simulink model "SUBS_PERFIL_OBSTACULOS"  (R2024b)
settings: Solver=VariableStepAuto  StartTime=0.0  StopTime=10.0  RelTol=1e-3
undefined symbols (not defined in the file): Wc
settings Model: Creator=juani  LastModifiedBy=juani

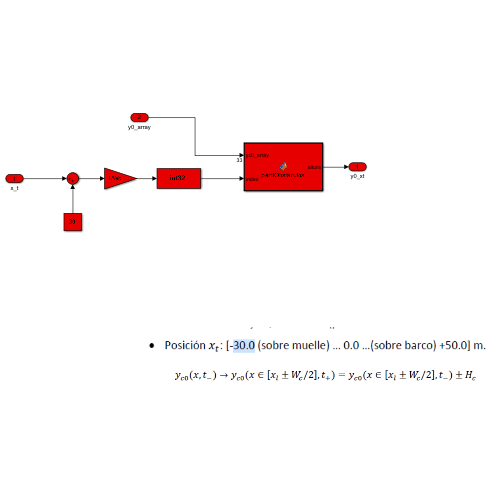
[thumbnail: Simulink's stored preview of the top-level diagram]
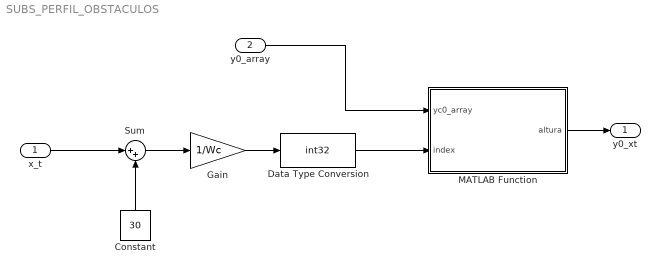
== system SUBS_PERFIL_OBSTACULOS ==
  x_t : Inport
  y0_array : Inport  Port=2
  Constant : Constant  Value=30
  Data Type Conversion : DataTypeConversion  OutDataTypeStr=int32  SaturateOnIntegerOverflow=off  RndMeth=Floor
  Gain : Gain  Gain=1/Wc
  MATLAB Function : MATLAB Function  TreatAsAtomicUnit=on
  Sum : Sum  Inputs=|++
  y0_xt : Outport
  wires:
  x_t/1 -> Sum/1
  Constant/1 -> Sum/2
  Sum/1 -> Gain/1
  y0_array/1 -> MATLAB Function/1(yc0_array)
  MATLAB Function/1(altura) -> y0_xt/1
  Gain/1 -> Data Type Conversion/1
  Data Type Conversion/1 -> MATLAB Function/2(index)

== matlab function SUBS_PERFIL_OBSTACULOS/MATLAB Function ==
  data: yc0_array input; altura output; index input
function altura = perfilObstaculos(yc0_array,index)

altura = yc0_array(index);
